simulink model "monteCarloTest"  (R2022b)
settings: Solver=FixedStepAuto  StartTime=0.0  StopTime=simParam.stopTime  FixedStep=simParam.maxStep  MaxStep=simParam.maxStep  RelTol=1e-3
undefined symbols (not defined in the file or in its folder): sigma, simParam
settings Model: Creator=kaike  LastModifiedBy=kaike

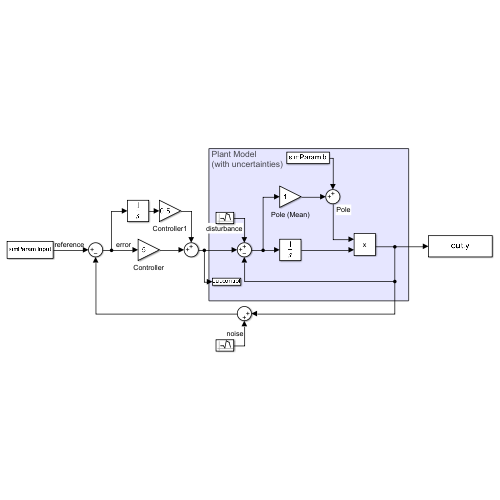
[thumbnail: Simulink's stored preview of the top-level diagram]
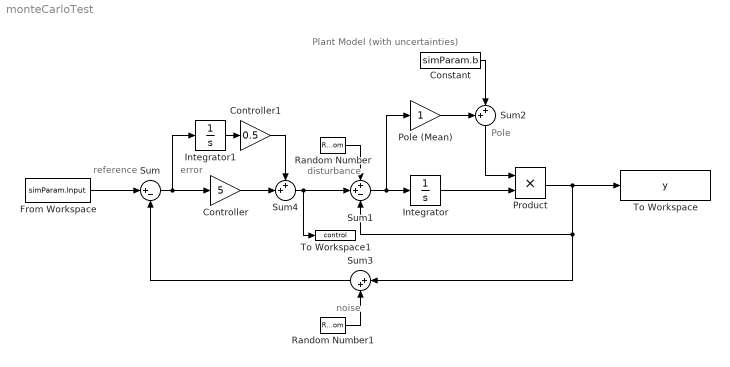
== system monteCarloTest ==
  note: noise
  note: disturbance
  note: error
  note: reference
  note: Pole
  note: Plant Model
      | (with uncertainties)
  Constant : Constant  Value=simParam.b
  Controller : Gain  Gain=5
  Controller1 : Gain  Gain=0.5
  From Workspace : FromWorkspace  VariableName=simParam.Input  OutputAfterFinalValue=Holding final value
  Integrator : Integrator
  Integrator1 : Integrator
  Pole (Mean) : Gain
  Product : Product
  Random Number : RandomNumber  Variance=sigma.d  Seed=simParam.seedDist
  Random Number1 : RandomNumber  Variance=sigma.n  Seed=simParam.seedNoise
  Sum : Sum  Inputs=|+-
  Sum1 : Sum  Inputs=++-
  Sum2 : Sum  Inputs=++|
  Sum3 : Sum  Inputs=|++
  Sum4 : Sum  Inputs=++|
  To Workspace : ToWorkspace  VariableName=y  SampleTime=-1
  To Workspace1 : ToWorkspace  VariableName=control  SampleTime=-1
  wires:
  Sum/1 -> Integrator1/1, Controller/1
  Sum1/1 -> Pole (Mean)/1, Integrator/1
  Integrator/1 -> Product/2
  Product/1 -> Sum3/1, Sum1/3, To Workspace/1
  Pole (Mean)/1 -> Sum2/1
  Sum2/1 -> Product/1
  Sum3/1 -> Sum/2
  From Workspace/1 -> Sum/1
  Constant/1 -> Sum2/2
  Random Number1/1 -> Sum3/2
  Random Number/1 -> Sum1/1
  Integrator1/1 -> Controller1/1
  Controller/1 -> Sum4/2
  Controller1/1 -> Sum4/1
  Sum4/1 -> To Workspace1/1, Sum1/2
